simulink model "outmodc_mdl"  (R2021b)
settings: Solver=ode1  StartTime=0.0  StopTime=100  FixedStep=0.001  MaxStep=0.1  MinStep=0.01  RelTol=1e-3
values from neighbouring files (symbols this model uses):
  A = A([2:end],[2:end])    [obsint_data.m]
  Am = A+B*Lx    [outmodc_data.m]
  B = B([2:end],:)    [obsint_data.m]
  Bm = B*-inv(Cm*inv(Am)*B)    [outmodc_data.m]
  C = C(:,:)    [obsint_data.m]
  rho = 1    [obsint_data.m]    (also in outmodc_data.m)
  S = rpp(Ai,Bi,Eopt)    [obsint_data.m]
  x0 = zeros(1,n)    [obsint_data.m]    (also in outmodc_data.m)
  xc0 = zeros(1,n-p)    [outmodc_data.m]
undefined symbols (not defined in the file or in its folder): Dhat, Hhat, L, Lam, Lr, Lx, m, n, p, P
settings Model: Creator=w.schwamm  LastModifiedBy=w.schwamm
settings DataIOCC: SaveOutput=off  SaveTime=off  ReturnWorkspaceOutputs=off  StateSaveName=x  TimeSaveName=t  OutputSaveName=y

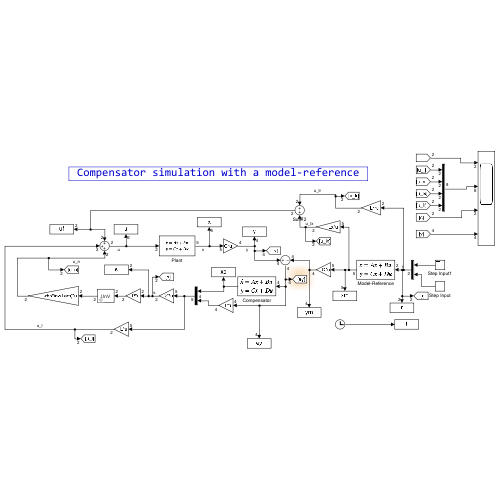
[thumbnail: Simulink's stored preview of the top-level diagram]
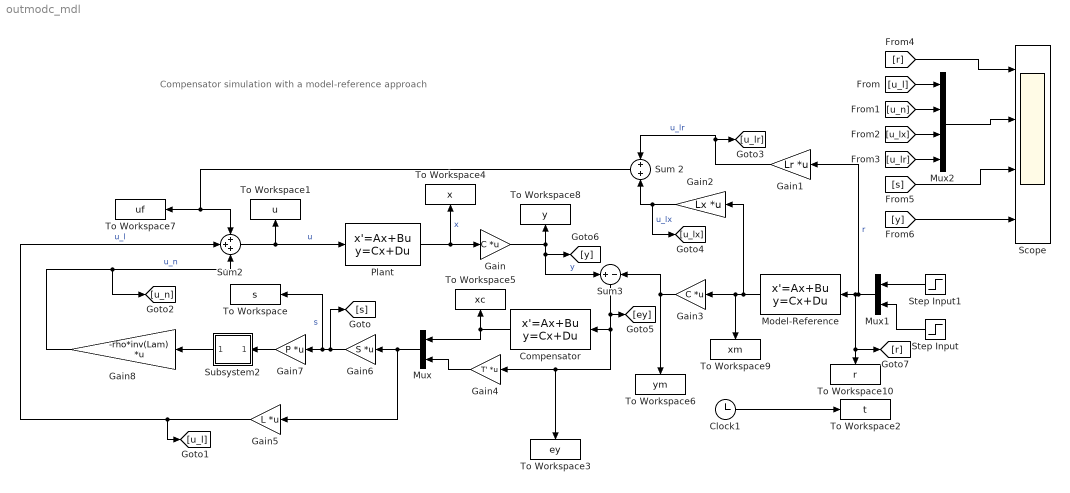
== system outmodc_mdl ==
  note: Compensator simulation with a model-reference approach
  Clock1 : Clock
  Compensator : StateSpace  A=Hhat  B=Dhat  C=eye(n-p)  D=zeros(n-p,p)  InitialCondition=xc0
  Gain : Gain  Gain=C  Multiplication=Matrix(K*u)
  Gain1 : Gain  Gain=Lr  Multiplication=Matrix(K*u)
  Gain2 : Gain  Gain=Lx  Multiplication=Matrix(K*u)
  Gain3 : Gain  Gain=C  Multiplication=Matrix(K*u)
  Gain4 : Gain  Gain=T'  Multiplication=Matrix(K*u)
  Gain5 : Gain  Gain=L  Multiplication=Matrix(K*u)
  Gain6 : Gain  Gain=S  Multiplication=Matrix(K*u)
  Gain7 : Gain  Gain=P  Multiplication=Matrix(K*u)
  Gain8 : Gain  Gain=-rho*inv(Lam)  Multiplication=Matrix(K*u)
  Model-Reference : StateSpace  A=Am  B=Bm  C=eye(n)  D=zeros(n,m)  InitialCondition=0
  Mux : Mux  Inputs=2
  Mux1 : Mux  Inputs=2
  Mux2 : Mux
  Plant : StateSpace  A=A  B=B  C=eye(n)  D=zeros(n,m)  InitialCondition=x0
  Scope : Scope  NumInputPorts=4
  Step Input : Step  Time=0  After=0.1  SampleTime=0
  Step Input1 : Step  Time=0  After=-0.25  SampleTime=0
  Subsystem2 : Subsystem  mask{delta=0.01}
      mask prompts: delta "Unit vector delta:"
      mask Display: disp('UnV')
  Sum 2 : Sum
  Sum2 : Sum  Inputs=+++
  Sum3 : Sum  Inputs=+-
  To Workspace : ToWorkspace  VariableName=s  SaveFormat=Timeseries  SampleTime=-1
      settings: MaxDataPoints=1000000
  To Workspace1 : ToWorkspace  VariableName=u  SaveFormat=Timeseries  SampleTime=-1
      settings: MaxDataPoints=1000000
  To Workspace10 : ToWorkspace  VariableName=r  SaveFormat=Timeseries  SampleTime=-1
      settings: MaxDataPoints=1000000
  To Workspace2 : ToWorkspace  VariableName=t  SaveFormat=Timeseries  SampleTime=-1
      settings: MaxDataPoints=1000000
  To Workspace3 : ToWorkspace  VariableName=ey  SaveFormat=Timeseries  SampleTime=-1
      settings: MaxDataPoints=1000000
  To Workspace4 : ToWorkspace  VariableName=x  SaveFormat=Timeseries  SampleTime=-1
      settings: MaxDataPoints=1000000
  To Workspace5 : ToWorkspace  VariableName=xc  SaveFormat=Timeseries  SampleTime=-1
      settings: MaxDataPoints=1000000
  To Workspace6 : ToWorkspace  VariableName=ym  SaveFormat=Timeseries  SampleTime=-1
      settings: MaxDataPoints=1000000
  To Workspace7 : ToWorkspace  VariableName=uf  SaveFormat=Timeseries  SampleTime=-1
      settings: MaxDataPoints=1000000
  To Workspace8 : ToWorkspace  VariableName=y  SaveFormat=Timeseries  SampleTime=-1
      settings: MaxDataPoints=1000000
  To Workspace9 : ToWorkspace  VariableName=xm  SaveFormat=Timeseries  SampleTime=-1
      settings: MaxDataPoints=1000000
  wires:
  Plant/1 -> Gain/1, To Workspace4/1  "x"
  Clock1/1 -> To Workspace2/1
  Sum2/1 -> To Workspace1/1, Plant/1  "u"
  Gain5/1 -> [u_l], Sum2/2  "u_l"
  Model-Reference/1 -> Gain2/1, Gain3/1, To Workspace9/1
  Gain/1 -> [y], Sum3/1, To Workspace8/1  "y"
  Gain3/1 -> Sum3/2, To Workspace6/1
  Sum3/1 -> [ey], Compensator/1, Gain4/1, To Workspace3/1
  Sum 2/1 -> Sum2/1, To Workspace7/1
  Subsystem2/1(Out1) -> Gain8/1
  Gain8/1 -> [u_n], Sum2/3  "u_n"
  Step Input1/1 -> Mux1/1
  Mux/1 -> Gain6/1, Gain5/1
  Gain4/1 -> Mux/2
  Compensator/1 -> Mux/1, To Workspace5/1
  Gain6/1 -> [s], Gain7/1, To Workspace/1  "s"
  Gain7/1 -> Subsystem2/1(In1)
  Mux1/1 -> Gain1/1, To Workspace10/1, [r], Model-Reference/1  "r"
  Step Input/1 -> Mux1/2
  Gain1/1 -> [u_lr], Sum 2/1  "u_lr"
  Gain2/1 -> [u_lx], Sum 2/2  "u_lx"
  [u_l] -> Mux2/1
  [u_n] -> Mux2/2
  [u_lx] -> Mux2/3
  [u_lr] -> Mux2/4
  [r] -> Scope/1
  Mux2/1 -> Scope/2
  [s] -> Scope/3
  [y] -> Scope/4

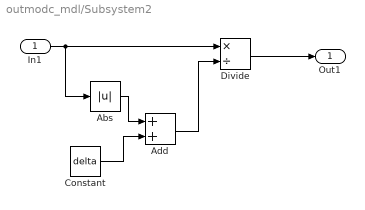
== system outmodc_mdl/Subsystem2 ==
  In1 : Inport
  Abs : Abs
  Add : Sum
  Constant : Constant  Value=delta  SampleTime=-1
  Divide : Product  Inputs=*/
  Out1 : Outport
  wires:
  Constant/1 -> Add/2
  Add/1 -> Divide/2
  Abs/1 -> Add/1
  Divide/1 -> Out1/1
  In1/1 -> Divide/1, Abs/1
